simulink model "linearmodelwithcontroller"  (R2016a)
settings: Solver=VariableStepAuto  StartTime=0.0  StopTime=100.0  RelTol=1e-3
libraries: simulink x2
settings Model: Creator=ASUS  LastModifiedBy=ASUS

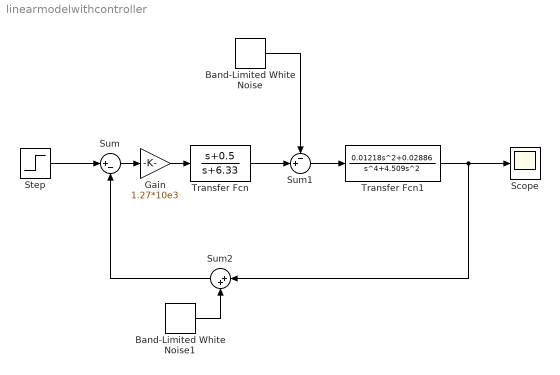
== system linearmodelwithcontroller ==
  Band-Limited White Noise : simulink/Sources/Band-Limited White Noise  Cov=10  Ts=0.1  seed=[23341]
  Band-Limited White Noise1 : simulink/Sources/Band-Limited White Noise  Cov=0.0001  Ts=0.1  seed=[23341]
  Gain : Gain  Gain=1.27*10e3
  Scope : Scope
  Step : Step  SampleTime=0
  Sum : Sum  Inputs=|+-
  Sum1 : Sum  Inputs=-+|
  Sum2 : Sum  Inputs=|++
  Transfer Fcn : TransferFcn  Numerator=[1 0.5]  Denominator=[1 6.33]
  Transfer Fcn1 : TransferFcn  Numerator=[0.01218 0 0.02886]  Denominator="[1 0  4.509 0 0 ]"
  wires:
  Step/1 -> Sum/1
  Sum1/1 -> Transfer Fcn1/1
  Transfer Fcn/1 -> Sum1/2
  Transfer Fcn1/1 -> Sum2/1, Scope/1
  Sum/1 -> Gain/1
  Gain/1 -> Transfer Fcn/1
  Band-Limited White Noise/1 -> Sum1/1
  Sum2/1 -> Sum/2
  Band-Limited White Noise1/1 -> Sum2/2
